simulink model "rsa_mwr2mm_core"  (R2021b)
settings: Solver=VariableStepAuto  StartTime=0.0  StopTime=simulation_time  RelTol=1e-3
values from neighbouring files (symbols this model uses):
  E = fi(hex2dec("4741"),0,max_n_bit,0)    [mwr2mm_init.m]    (also in rsa_mwr2mm_init.m)
  K = fi(mod((4)^max_n_bit,double(N)),0,max_n_bit,0)    [mwr2mm_init.m]    (also in rsa_mwr2mm_init.m)
  M = fi(hex2dec("2f76"),0,max_n_bit,0)    [mwr2mm_init.m]    (also in rsa_mwr2mm_init.m)
  max_n_bit = 16    [mwr2mm_init.m]    (also in rsa_mwr2mm_init.m)
  N = fi(hex2dec("8167"),0,max_n_bit,0)    [mwr2mm_init.m]    (also in rsa_mwr2mm_init.m)
  number_of_pe = ceil((max_n_bit+1)/word_length)    [mwr2mm_init.m]    (also in rsa_mwr2mm_init.m)
  ts = 1/fs    (= 4e-09)    [mwr2mm_init.m]    (also in rsa_mwr2mm_init.m)
  word_length = 4    [mwr2mm_init.m]    (also in rsa_mwr2mm_init.m)
libraries: xbsIndex_r4 x206
(part 1 of 2)
settings Model: Creator=HosseinBehehsti  LastModifiedBy=sysgen

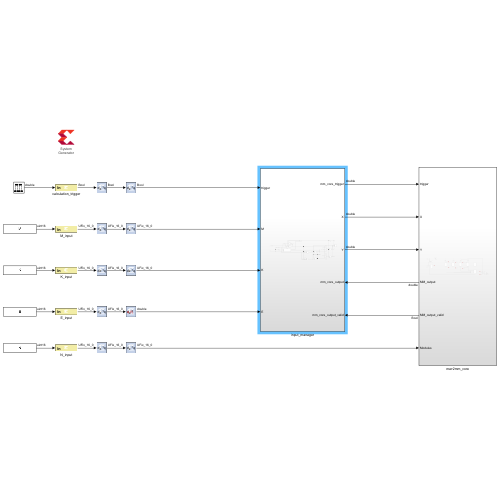
[thumbnail: Simulink's stored preview of the top-level diagram]
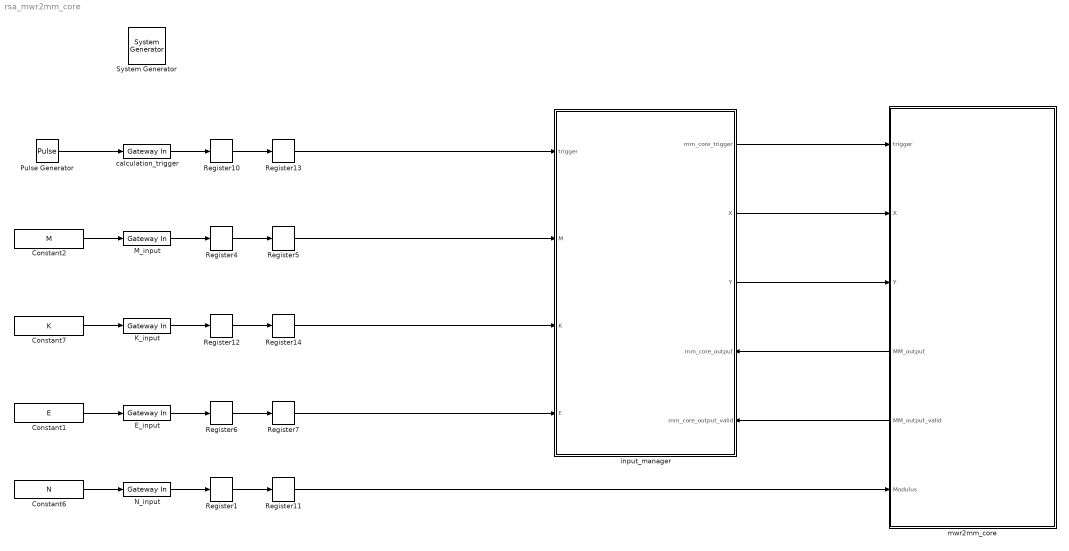
== system rsa_mwr2mm_core ==
  " System Generator" : xbsIndex_r4/ System Generator  Tag=genX  xilinxfamily=kintex7  part=xc7k325t  speed=-2  package=ffg676  synthesis_tool=Vivado  clock_wrapper=Clock Enables  directory=./netlist  proj_type=Vivado  Synth_file=Vivado Synthesis Defaults  Impl_file=Vivado Implementation Defaults  testbench=off  simulink_period=ts  sysclk_period=ts*1e9  dcm_input_clock_period=10  incr_netlist=off  trim_vbits=Everywhere in SubSystem  dbl_ovrd=According to Block Masks  core_generation=According to Block Masks  run_coregen=off  deprecated_control=off  eval_field=0  block_type=sysgen
  Constant1 : Constant  Value=E
  Constant2 : Constant  Value=M
  Constant6 : Constant  Value=N
  Constant7 : Constant  Value=K
  E_input : xbsIndex_r4/Gateway In  gui_display_data_type=Fixed-point  arith_type=Unsigned  n_bits=max_n_bit  bin_pt=0  preci_type=Single  exp_width=8  frac_width=24  rows=1  columns=1  quantization="Round  (unbiased: +/- Inf)"  overflow=Saturate  period=ts  UseAsADC=off  ADCChannel='1'  interface=None  automatic_assignment=on  address_offset=hex2dec('00')  intf_name=''  intf_description=''  default_value=0  timing_constraint=None  locs_specified=off  LOCs={}  io_standard={}  inherit_from_input=off  hdl_port=on  dbl_ovrd=off  block_type=gatewayin
  K_input : xbsIndex_r4/Gateway In  gui_display_data_type=Fixed-point  arith_type=Unsigned  n_bits=max_n_bit  bin_pt=0  preci_type=Single  exp_width=8  frac_width=24  rows=1  columns=1  quantization="Round  (unbiased: +/- Inf)"  overflow=Saturate  period=ts  UseAsADC=off  ADCChannel='1'  interface=None  automatic_assignment=on  address_offset=hex2dec('00')  intf_name=''  intf_description=''  default_value=0  timing_constraint=None  locs_specified=off  LOCs={}  io_standard={}  inherit_from_input=off  hdl_port=on  dbl_ovrd=off  block_type=gatewayin
  M_input : xbsIndex_r4/Gateway In  gui_display_data_type=Fixed-point  arith_type=Unsigned  n_bits=max_n_bit  bin_pt=0  preci_type=Single  exp_width=8  frac_width=24  rows=1  columns=1  quantization="Round  (unbiased: +/- Inf)"  overflow=Saturate  period=ts  UseAsADC=off  ADCChannel='1'  interface=None  automatic_assignment=on  address_offset=hex2dec('00')  intf_name=''  intf_description=''  default_value=0  timing_constraint=None  locs_specified=off  LOCs={}  io_standard={}  inherit_from_input=off  hdl_port=on  dbl_ovrd=off  block_type=gatewayin
  N_input : xbsIndex_r4/Gateway In  gui_display_data_type=Fixed-point  arith_type=Unsigned  n_bits=max_n_bit  bin_pt=0  preci_type=Single  exp_width=8  frac_width=24  rows=1  columns=1  quantization="Round  (unbiased: +/- Inf)"  overflow=Saturate  period=ts  UseAsADC=off  ADCChannel='1'  interface=None  automatic_assignment=on  address_offset=hex2dec('00')  intf_name=''  intf_description=''  default_value=0  timing_constraint=None  locs_specified=off  LOCs={}  io_standard={}  inherit_from_input=off  hdl_port=on  dbl_ovrd=off  block_type=gatewayin
  Pulse Generator : DiscretePulseGenerator  Period=10000  PhaseDelay=30  SampleTime=ts
  Register{1,4..7,10..14} (10 alike) : xbsIndex_r4/Register  init=0  rst=off  en=off  dbl_ovrd=off  block_type=register
  calculation_trigger : xbsIndex_r4/Gateway In  gui_display_data_type=Boolean  arith_type=Boolean  n_bits=16  bin_pt=14  preci_type=Single  exp_width=8  frac_width=24  rows=1  columns=1  quantization="Round  (unbiased: +/- Inf)"  overflow=Saturate  period=ts  UseAsADC=off  ADCChannel='1'  interface=None  automatic_assignment=on  address_offset=hex2dec('00')  intf_name=''  intf_description=''  default_value=0  timing_constraint=None  locs_specified=off  LOCs={}  io_standard={}  inherit_from_input=off  hdl_port=on  dbl_ovrd=off  block_type=gatewayin
  input_manager : Subsystem
      settings: PortSchema="{\"entries\":[{\"content\":{\"sides\":[{\"content\":{\"connectorIds\":[\"In1\",\"In2\",\"In3\",\"In4\"]},\"type\":\"ConnectorPlacement.EquallySpacedRectSide\",\"uuid\":\"5fbe749b-9735-44fd-a2bb-776500a26cf7\"},{\"content\":{\"connectorIds\":[\"Out1\",\"Out2\",\"Out3\",\"In5\",\"In6\"],\"side\":\"RIGHT\"},\"type\":\"ConnectorPlacement.EquallySpacedRectSide\",\"uuid\":\"76eb6fff-7389-4eb3-99ce-2472142167d3\"},{\"content\":{\"connectorIds\":[],\"side\":\"TOP\"},\"type\":\"ConnectorPlacement.EquallySpacedRectSide\",\"uuid\":\"3dd7521d-ec81-483b-a940-2bc8a970d0b7\"}]},\"type\":\"ConnectorPlacement.EquallySpacedConnector\",\"uuid\":\"ad526796-1480-458f-ab98-8695681b9dff\"}],\"packageUris\":[\"http://schema.mathworks.com/mf0/Connector/R2020b\"],\"version\":\"1.0\"}"
  mwr2mm_core : Subsystem
      settings: PortSchema="{\"entries\":[{\"content\":{\"sides\":[{\"content\":{\"connectorIds\":[\"In1\",\"In2\",\"In3\",\"Out1\",\"Out2\",\"In4\"]},\"type\":\"ConnectorPlacement.EquallySpacedRectSide\",\"uuid\":\"3849742e-47e7-45e9-813d-75e7ec89f679\"},{\"content\":{\"connectorIds\":[],\"side\":\"RIGHT\"},\"type\":\"ConnectorPlacement.EquallySpacedRectSide\",\"uuid\":\"56ecc40d-88ec-4579-a1b5-d15bded2ad6c\"},{\"content\":{\"connectorIds\":[],\"side\":\"TOP\"},\"type\":\"ConnectorPlacement.EquallySpacedRectSide\",\"uuid\":\"95912069-9c19-4eb9-99de-47b6cc07ccbf\"}]},\"type\":\"ConnectorPlacement.EquallySpacedConnector\",\"uuid\":\"0eef9a1f-cfa8-4a5c-bd29-08fde97e02e9\"}],\"packageUris\":[\"http://schema.mathworks.com/mf0/Connector/R2020b\"],\"version\":\"1.0\"}"
  wires:
  Register4/1 -> Register5/1
  M_input/1 -> Register4/1
  E_input/1 -> Register6/1
  Register6/1 -> Register7/1
  Register10/1 -> Register13/1
  calculation_trigger/1 -> Register10/1
  Constant1/1 -> E_input/1
  Constant2/1 -> M_input/1
  Pulse Generator/1 -> calculation_trigger/1
  Constant6/1 -> N_input/1
  Register1/1 -> Register11/1
  N_input/1 -> Register1/1
  K_input/1 -> Register12/1
  Register12/1 -> Register14/1
  Constant7/1 -> K_input/1
  Register11/1 -> mwr2mm_core/4(Modulus)
  Register5/1 -> input_manager/2(M)
  Register14/1 -> input_manager/3(K)
  input_manager/2(X) -> mwr2mm_core/2(X)
  input_manager/3(Y) -> mwr2mm_core/3(Y)
  Register13/1 -> input_manager/1(trigger)
  Register7/1 -> input_manager/4(E)
  input_manager/1(mm_core_trigger) -> mwr2mm_core/1(trigger)
  mwr2mm_core/1(MM_output) -> input_manager/5(mm_core_output)
  mwr2mm_core/2(MM_output_valid) -> input_manager/6(mm_core_output_valid)

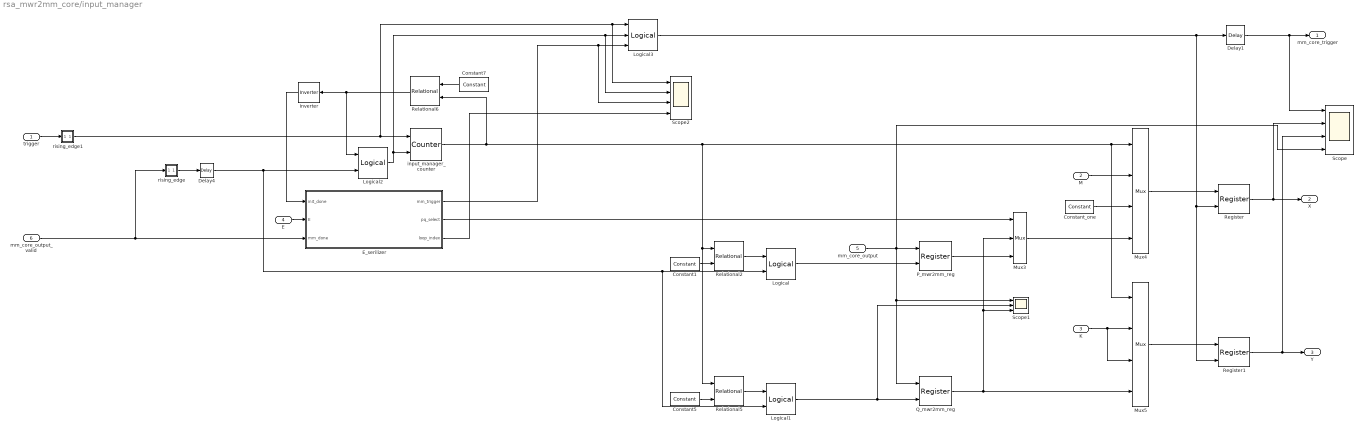
== system rsa_mwr2mm_core/input_manager ==
  trigger : Inport
  M : Inport  Port=2
  K : Inport  Port=3
  E : Inport  Port=4
  mm_core_output : Inport  Port=5
  mm_core_output_valid : Inport  Port=6
  Constant1 : xbsIndex_r4/Constant  const=0  gui_display_data_type=Fixed-point  arith_type=Unsigned  n_bits=2  bin_pt=0  preci_type=Single  exp_width=8  frac_width=24  explicit_period=off  period=1  equ=P=C  opselect=C  inp2=PCIN>>17  opr=+  inp1=P  carry=CIN  dbl_ovrd=off  block_type=constant
  Constant5 : xbsIndex_r4/Constant  const=0  gui_display_data_type=Fixed-point  arith_type=Unsigned  n_bits=2  bin_pt=0  preci_type=Single  exp_width=8  frac_width=24  explicit_period=off  period=1  equ=P=C  opselect=C  inp2=PCIN>>17  opr=+  inp1=P  carry=CIN  dbl_ovrd=off  block_type=constant
  Constant7 : xbsIndex_r4/Constant  const=2  gui_display_data_type=Fixed-point  arith_type=Unsigned  n_bits=2  bin_pt=0  preci_type=Single  exp_width=8  frac_width=24  explicit_period=off  period=1  equ=P=C  opselect=C  inp2=PCIN>>17  opr=+  inp1=P  carry=CIN  dbl_ovrd=off  block_type=constant
  Constant_one : xbsIndex_r4/Constant  const=1.0  gui_display_data_type=Fixed-point  arith_type=Unsigned  n_bits=max_n_bit  bin_pt=0  preci_type=Single  exp_width=8  frac_width=24  explicit_period=off  period=1  equ=P=C  opselect=C  inp2=PCIN>>17  opr=+  inp1=P  carry=CIN  dbl_ovrd=off  block_type=constant
  Delay1 : xbsIndex_r4/Delay  rst=off  infoeditControl=Selection of Reset will increase slice count due to use of real FFs and instead of SRLs  en=off  latency=4  reg_retiming=off  dbl_ovrd=off  block_type=delay
  Delay4 : xbsIndex_r4/Delay  rst=off  infoeditControl=Selection of Reset will increase slice count due to use of real FFs and instead of SRLs  en=off  latency=11  reg_retiming=off  dbl_ovrd=off  block_type=delay
  E_serilizer : Subsystem
  Inverter : xbsIndex_r4/Inverter  en=off  latency=1  dbl_ovrd=off  block_type=inv
  Logical : xbsIndex_r4/Logical  logical_function=AND  inputs=2  en=off  latency=1  precision=Full  arith_type=Unsigned  n_bits=16  bin_pt=0  align_bp=on  dbl_ovrd=off  block_type=logical
  Logical1 : xbsIndex_r4/Logical  logical_function=AND  inputs=2  en=off  latency=1  precision=Full  arith_type=Unsigned  n_bits=16  bin_pt=0  align_bp=on  dbl_ovrd=off  block_type=logical
  Logical2 : xbsIndex_r4/Logical  logical_function=AND  inputs=2  en=off  latency=0  precision=Full  arith_type=Unsigned  n_bits=16  bin_pt=0  align_bp=on  dbl_ovrd=off  block_type=logical
  Logical3 : xbsIndex_r4/Logical  logical_function=OR  inputs=3  en=off  latency=0  precision=Full  arith_type=Unsigned  n_bits=16  bin_pt=0  align_bp=on  dbl_ovrd=off  block_type=logical
  Mux3 : xbsIndex_r4/Mux  inputs=2  en=off  latency=0  precision=Full  arith_type=Unsigned  n_bits=16  bin_pt=14  quantization=Truncate  overflow=Wrap  dbl_ovrd=off  block_type=mux
  Mux4 : xbsIndex_r4/Mux  inputs=3  en=off  latency=1  precision=Full  arith_type=Unsigned  n_bits=16  bin_pt=14  quantization=Truncate  overflow=Wrap  dbl_ovrd=off  block_type=mux
  Mux5 : xbsIndex_r4/Mux  inputs=3  en=off  latency=1  precision=Full  arith_type=Unsigned  n_bits=16  bin_pt=14  quantization=Truncate  overflow=Wrap  dbl_ovrd=off  block_type=mux
  P_mwr2mm_reg : xbsIndex_r4/Register  init=0  rst=off  en=on  dbl_ovrd=off  block_type=register
  Q_mwr2mm_reg : xbsIndex_r4/Register  init=0  rst=off  en=on  dbl_ovrd=off  block_type=register
  Register : xbsIndex_r4/Register  init=0  rst=off  en=on  dbl_ovrd=off  block_type=register
  Register1 : xbsIndex_r4/Register  init=0  rst=off  en=on  dbl_ovrd=off  block_type=register
  Relational2 : xbsIndex_r4/Relational  mode=a=b  op_type=Bool  en=off  latency=0  dbl_ovrd=off  block_type=relational
  Relational5 : xbsIndex_r4/Relational  mode=a!=b  op_type=Bool  en=off  latency=0  dbl_ovrd=off  block_type=relational
  Relational6 : xbsIndex_r4/Relational  mode=a!=b  op_type=Bool  en=off  latency=0  dbl_ovrd=off  block_type=relational
  Scope : Scope  NumInputPorts=4
  Scope1 : Scope  NumInputPorts=3
  Scope2 : Scope  NumInputPorts=4
  input_manager_counter : xbsIndex_r4/Counter  cnt_type=Count Limited  cnt_to=2  operation=Up  start_count=0  cnt_by_val=1  arith_type=Unsigned  n_bits=2  bin_pt=0  load_pin=off  rst=on  en=on  explicit_period=off  period=1  use_behavioral_HDL=off  implementation=Fabric  dbl_ovrd=off  block_type=counter
  rising_edge : Subsystem
  rising_edge1 : Subsystem
  mm_core_trigger : Outport
  X : Outport  Port=2
  Y : Outport  Port=3
  wires:
  E_serilizer/2(pq_select) -> Mux3/1
  Q_mwr2mm_reg/1 -> Mux5/4, Scope1/3, Mux3/2
  P_mwr2mm_reg/1 -> Mux3/3
  mm_core_output/1 -> Q_mwr2mm_reg/1, Scope1/1, Scope/4, P_mwr2mm_reg/1
  mm_core_output_valid/1 -> rising_edge/1(input), E_serilizer/3(mm_done)
  Relational2/1 -> Logical/1
  Constant1/1 -> Relational2/2
  Logical/1 -> P_mwr2mm_reg/2
  trigger/1 -> rising_edge1/1(input)
  rising_edge1/1(redge) -> Scope2/1, Logical3/1, input_manager_counter/1
  E_serilizer/1(mm_trigger) -> Scope2/3, Logical3/3
  Constant5/1 -> Relational5/2
  Relational5/1 -> Logical1/1
  Logical1/1 -> Scope1/2, Q_mwr2mm_reg/2
  E/1 -> E_serilizer/2(E)
  Constant7/1 -> Relational6/1
  Logical2/1 -> Scope2/2, Logical3/2, input_manager_counter/2
  Relational6/1 -> Logical2/1, Inverter/1
  Inverter/1 -> E_serilizer/1(init_done)
  input_manager_counter/1 -> Relational6/2, Mux5/1, Mux4/1, Relational5/1, Relational2/1
  rising_edge/1(redge) -> Delay4/1
  Delay4/1 -> Logical2/2, Logical1/2, Logical/2
  Register/1 -> Scope/2, X/1
  Register1/1 -> Scope/3, Y/1
  Delay1/1 -> Scope/1, mm_core_trigger/1
  M/1 -> Mux4/2
  Mux4/1 -> Register/1
  Mux5/1 -> Register1/1
  K/1 -> Mux5/3, Mux5/2
  Constant_one/1 -> Mux4/3
  Mux3/1 -> Mux4/4
  Logical3/1 -> Register/2, Register1/2, Delay1/1
  E_serilizer/3(loop_index) -> Scope2/4

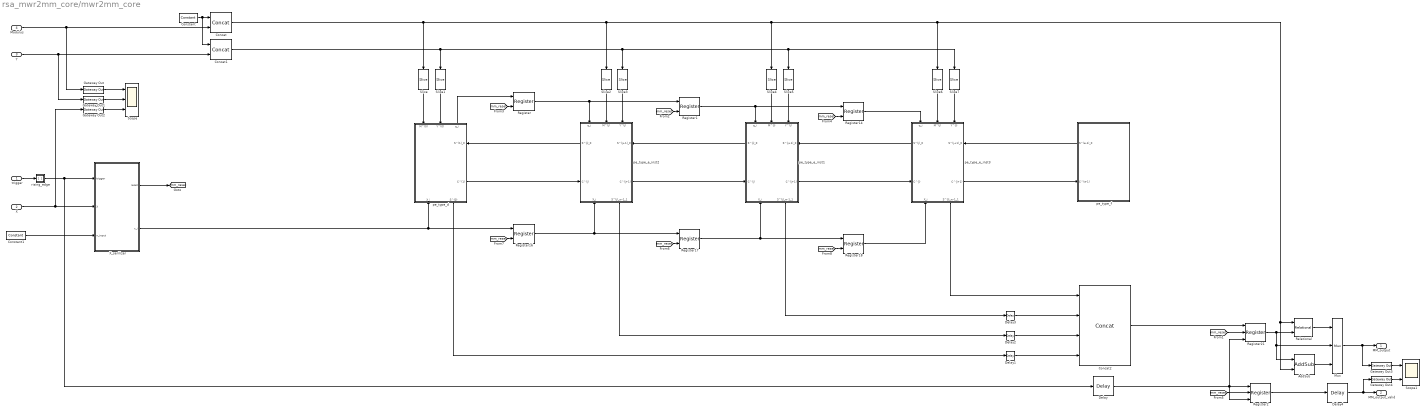
== system rsa_mwr2mm_core/mwr2mm_core ==
  trigger : Inport
  X : Inport  Port=2
  Y : Inport  Port=3
  Modulus : Inport  Port=4
  AddSub : xbsIndex_r4/AddSub  mode=Subtraction  use_carryin=off  use_carryout=off  en=off  latency=1  precision=User Defined  arith_type=Unsigned  n_bits=max_n_bit  bin_pt=0  quantization="Round  (unbiased: +/- Inf)"  overflow=Saturate  use_behavioral_HDL=off  hw_selection=Fabric  pipelined=off  dbl_ovrd=off  block_type=addsub
  Concat : xbsIndex_r4/Concat  num_inputs=2  dbl_ovrd=off  block_type=concat
  Concat1 : xbsIndex_r4/Concat  num_inputs=2  dbl_ovrd=off  block_type=concat
  Concat2 : xbsIndex_r4/Concat  num_inputs=4  dbl_ovrd=off  block_type=concat
  Constant : xbsIndex_r4/Constant  const=0  gui_display_data_type=Fixed-point  arith_type=Unsigned  n_bits=word_length  bin_pt=0  preci_type=Single  exp_width=8  frac_width=24  explicit_period=off  period=1  equ=P=C  opselect=C  inp2=PCIN>>17  opr=+  inp1=P  carry=CIN  dbl_ovrd=off  block_type=constant
  Constant1 : xbsIndex_r4/Constant  const=max_n_bit-1  gui_display_data_type=Fixed-point  arith_type=Unsigned  n_bits=ceil(log2(max_n_bit))  bin_pt=0  preci_type=Single  exp_width=8  frac_width=24  explicit_period=on  period=ts  equ=P=C  opselect=C  inp2=PCIN>>17  opr=+  inp1=P  carry=CIN  dbl_ovrd=off  block_type=constant
  Delay : xbsIndex_r4/Delay  rst=off  infoeditControl=Selection of Reset will increase slice count due to use of real FFs and instead of SRLs  en=off  latency=max_n_bit+number_of_pe+5  reg_retiming=off  dbl_ovrd=off  block_type=delay
  Delay1 : xbsIndex_r4/Delay  rst=off  infoeditControl=Selection of Reset will increase slice count due to use of real FFs and instead of SRLs  en=off  latency=3  reg_retiming=off  dbl_ovrd=off  block_type=delay
  Delay2 : xbsIndex_r4/Delay  rst=off  infoeditControl=Selection of Reset will increase slice count due to use of real FFs and instead of SRLs  en=off  latency=2  reg_retiming=off  dbl_ovrd=off  block_type=delay
  Delay3 : xbsIndex_r4/Delay  rst=off  infoeditControl=Selection of Reset will increase slice count due to use of real FFs and instead of SRLs  en=off  latency=1  reg_retiming=off  dbl_ovrd=off  block_type=delay
  Delay4 : xbsIndex_r4/Delay  rst=off  infoeditControl=Selection of Reset will increase slice count due to use of real FFs and instead of SRLs  en=off  latency=3  reg_retiming=off  dbl_ovrd=off  block_type=delay
  Gateway Out{,1..4} (5 alike) : xbsIndex_r4/Gateway Out  inherit_from_input=off  hdl_port=off  rows=1  columns=1  UseAsDAC=off  DACChannel='1'  interface=None  automatic_assignment=on  address_offset=hex2dec('00')  intf_name=''  intf_description=''  timing_constraint=None  locs_specified=off  LOCs={}  io_standard={}  block_type=gatewayout
  Mux : xbsIndex_r4/Mux  inputs=2  en=off  latency=1  precision=Full  arith_type=Unsigned  n_bits=16  bin_pt=14  quantization=Truncate  overflow=Wrap  dbl_ovrd=off  block_type=mux
  Register{,1,14,16..18} (6 alike) : xbsIndex_r4/Register  init=0  rst=on  en=off  dbl_ovrd=off  block_type=register
  Register2 : xbsIndex_r4/Register  init=0  rst=on  en=on  dbl_ovrd=off  block_type=register
  Register21 : xbsIndex_r4/Register  init=0  rst=on  en=on  dbl_ovrd=off  block_type=register
  Relational : xbsIndex_r4/Relational  mode=a<b  op_type=Bool  en=off  latency=1  dbl_ovrd=off  block_type=relational
  Scope : Scope  NumInputPorts=3
  Scope1 : Scope  NumInputPorts=2
  Slice : xbsIndex_r4/Slice  nbits=word_length  boolean_output=off  mode=Lower Bit Location + Width  bit1=0  base1=MSB of Input  bit0=0  base0=LSB of Input  dbl_ovrd=off  block_type=slice
  Slice1 : xbsIndex_r4/Slice  nbits=word_length  boolean_output=off  mode=Lower Bit Location + Width  bit1=0  base1=MSB of Input  bit0=0  base0=LSB of Input  dbl_ovrd=off  block_type=slice
  Slice2 : xbsIndex_r4/Slice  nbits=word_length  boolean_output=off  mode=Lower Bit Location + Width  bit1=0  base1=MSB of Input  bit0=1*word_length  base0=LSB of Input  dbl_ovrd=off  block_type=slice
  Slice3 : xbsIndex_r4/Slice  nbits=word_length  boolean_output=off  mode=Lower Bit Location + Width  bit1=0  base1=MSB of Input  bit0=1*word_length  base0=LSB of Input  dbl_ovrd=off  block_type=slice
  Slice4 : xbsIndex_r4/Slice  nbits=word_length  boolean_output=off  mode=Lower Bit Location + Width  bit1=0  base1=MSB of Input  bit0=2*word_length  base0=LSB of Input  dbl_ovrd=off  block_type=slice
  Slice5 : xbsIndex_r4/Slice  nbits=word_length  boolean_output=off  mode=Lower Bit Location + Width  bit1=0  base1=MSB of Input  bit0=2*word_length  base0=LSB of Input  dbl_ovrd=off  block_type=slice
  Slice6 : xbsIndex_r4/Slice  nbits=word_length  boolean_output=off  mode=Lower Bit Location + Width  bit1=0  base1=MSB of Input  bit0=3*word_length  base0=LSB of Input  dbl_ovrd=off  block_type=slice
  Slice7 : xbsIndex_r4/Slice  nbits=word_length  boolean_output=off  mode=Lower Bit Location + Width  bit1=0  base1=MSB of Input  bit0=3*word_length  base0=LSB of Input  dbl_ovrd=off  block_type=slice
  X_serilizer : Subsystem
  pe_type_d : Subsystem
      settings: PortSchema="{\"entries\":[{\"content\":{\"sides\":[{\"content\":{\"connectorIds\":[]},\"type\":\"ConnectorPlacement.EquallySpacedRectSide\",\"uuid\":\"139fe22c-bad5-4a8c-bb4f-0e4abe8a2134\"},{\"content\":{\"connectorIds\":[\"In4\",\"Out1\"],\"side\":\"RIGHT\"},\"type\":\"ConnectorPlacement.EquallySpacedRectSide\",\"uuid\":\"0caa1206-8436-46b5-be2a-5ee3acf33157\"},{\"content\":{\"connectorIds\":[\"In1\",\"In2\",\"Out3\"],\"side\":\"TOP\"},\"type\":\"ConnectorPlacement.EquallySpacedRectSide\",\"uuid\":\"0f19409c-37a1-4e1f-8a36-d56d656a29ed\"},{\"content\":{\"connectorIds\":[\"In3\",\"Out2\"],\"side\":\"BOTTOM\"},\"type\":\"ConnectorPlacement.EquallySpacedRectSide\",\"uuid\":\"3eb4fdbb-82ed-4bb4-bb3d-1ea670375199\"}]},\"type\":\"ConnectorPlacement.EquallySpacedConnector\",\"uuid\":\"2e2112f8-b3e9-4cf9-af24-9d5d119acc0c\"}],\"packageUris\":[\"http://schema.mathworks.com/mf0/Connector/R2020b\"],\"version\":\"1.0\"}"
  pe_type_e_inst1 : Subsystem
      settings: PortSchema="{\"entries\":[{\"content\":{\"sides\":[{\"content\":{\"connectorIds\":[\"Out3\",\"In1\"]},\"type\":\"ConnectorPlacement.EquallySpacedRectSide\",\"uuid\":\"7c8435b2-413b-47b3-86e2-fbe621383b46\"},{\"content\":{\"connectorIds\":[\"In6\",\"Out1\"],\"side\":\"RIGHT\"},\"type\":\"ConnectorPlacement.EquallySpacedRectSide\",\"uuid\":\"f6a32e17-79c6-4fcd-9120-5459a6da7349\"},{\"content\":{\"connectorIds\":[\"In2\",\"In3\",\"In4\"],\"side\":\"TOP\"},\"type\":\"ConnectorPlacement.EquallySpacedRectSide\",\"uuid\":\"72801329-e094-46db-be09-4f98df807717\"},{\"content\":{\"connectorIds\":[\"In5\",\"Out2\"],\"side\":\"BOTTOM\"},\"type\":\"ConnectorPlacement.EquallySpacedRectSide\",\"uuid\":\"81172500-9a38-48f4-98da-a2165838752d\"}]},\"type\":\"ConnectorPlacement.EquallySpacedConnector\",\"uuid\":\"de64cd8a-ab75-41df-a3d4-83ece8cdbbe2\"}],\"packageUris\":[\"http://schema.mathworks.com/mf0/Connector/R2020b\"],\"version\":\"1.0\"}"
  pe_type_e_inst2 : Subsystem
      settings: PortSchema="{\"entries\":[{\"content\":{\"sides\":[{\"content\":{\"connectorIds\":[\"Out3\",\"In1\"]},\"type\":\"ConnectorPlacement.EquallySpacedRectSide\",\"uuid\":\"7c8435b2-413b-47b3-86e2-fbe621383b46\"},{\"content\":{\"connectorIds\":[\"In6\",\"Out1\"],\"side\":\"RIGHT\"},\"type\":\"ConnectorPlacement.EquallySpacedRectSide\",\"uuid\":\"f6a32e17-79c6-4fcd-9120-5459a6da7349\"},{\"content\":{\"connectorIds\":[\"In2\",\"In3\",\"In4\"],\"side\":\"TOP\"},\"type\":\"ConnectorPlacement.EquallySpacedRectSide\",\"uuid\":\"72801329-e094-46db-be09-4f98df807717\"},{\"content\":{\"connectorIds\":[\"In5\",\"Out2\"],\"side\":\"BOTTOM\"},\"type\":\"ConnectorPlacement.EquallySpacedRectSide\",\"uuid\":\"81172500-9a38-48f4-98da-a2165838752d\"}]},\"type\":\"ConnectorPlacement.EquallySpacedConnector\",\"uuid\":\"de64cd8a-ab75-41df-a3d4-83ece8cdbbe2\"}],\"packageUris\":[\"http://schema.mathworks.com/mf0/Connector/R2020b\"],\"version\":\"1.0\"}"
  pe_type_e_inst3 : Subsystem
      settings: PortSchema="{\"entries\":[{\"content\":{\"sides\":[{\"content\":{\"connectorIds\":[\"Out3\",\"In1\"]},\"type\":\"ConnectorPlacement.EquallySpacedRectSide\",\"uuid\":\"7c8435b2-413b-47b3-86e2-fbe621383b46\"},{\"content\":{\"connectorIds\":[\"In6\",\"Out1\"],\"side\":\"RIGHT\"},\"type\":\"ConnectorPlacement.EquallySpacedRectSide\",\"uuid\":\"f6a32e17-79c6-4fcd-9120-5459a6da7349\"},{\"content\":{\"connectorIds\":[\"In2\",\"In3\",\"In4\"],\"side\":\"TOP\"},\"type\":\"ConnectorPlacement.EquallySpacedRectSide\",\"uuid\":\"72801329-e094-46db-be09-4f98df807717\"},{\"content\":{\"connectorIds\":[\"In5\",\"Out2\"],\"side\":\"BOTTOM\"},\"type\":\"ConnectorPlacement.EquallySpacedRectSide\",\"uuid\":\"81172500-9a38-48f4-98da-a2165838752d\"}]},\"type\":\"ConnectorPlacement.EquallySpacedConnector\",\"uuid\":\"de64cd8a-ab75-41df-a3d4-83ece8cdbbe2\"}],\"packageUris\":[\"http://schema.mathworks.com/mf0/Connector/R2020b\"],\"version\":\"1.0\"}"
  pe_type_f : Subsystem
      settings: PortSchema="{\"entries\":[{\"content\":{\"sides\":[{\"content\":{\"connectorIds\":[\"Out1\",\"In1\"]},\"type\":\"ConnectorPlacement.EquallySpacedRectSide\",\"uuid\":\"7c8435b2-413b-47b3-86e2-fbe621383b46\"},{\"content\":{\"connectorIds\":[],\"side\":\"RIGHT\"},\"type\":\"ConnectorPlacement.EquallySpacedRectSide\",\"uuid\":\"f6a32e17-79c6-4fcd-9120-5459a6da7349\"},{\"content\":{\"connectorIds\":[],\"side\":\"TOP\"},\"type\":\"ConnectorPlacement.EquallySpacedRectSide\",\"uuid\":\"72801329-e094-46db-be09-4f98df807717\"},{\"content\":{\"connectorIds\":[],\"side\":\"BOTTOM\"},\"type\":\"ConnectorPlacement.EquallySpacedRectSide\",\"uuid\":\"86ccfa13-264b-4b98-8cad-be21ce563201\"}]},\"type\":\"ConnectorPlacement.EquallySpacedConnector\",\"uuid\":\"de64cd8a-ab75-41df-a3d4-83ece8cdbbe2\"}],\"packageUris\":[\"http://schema.mathworks.com/mf0/Connector/R2020b\"],\"version\":\"1.0\"}"
  rising_edge : Subsystem
  MM_output : Outport
  MM_output_valid : Outport  Port=2
  tag scope: mm_reset=global
  wires:
  pe_type_d/2(S^(0)) -> Delay1/1
  [mm_reset] -> Register14/2
  pe_type_e_inst1/1(C^(j+1)) -> pe_type_e_inst3/1(C^(j))
  pe_type_d/1(C^(1)) -> pe_type_e_inst2/1(C^(j))
  Register16/1 -> pe_type_e_inst2/5(X_i), Register17/1
  Delay3/1 -> Concat2/2
  Register17/1 -> pe_type_e_inst1/5(X_i), Register18/1
  Register18/1 -> pe_type_e_inst3/5(X_i)
  Concat/1 -> Slice/1, Slice2/1, Slice4/1, Slice6/1, AddSub/2, Relational/1
  pe_type_e_inst2/1(C^(j+1)) -> pe_type_e_inst1/1(C^(j))
  X_serilizer/2(x_i) -> pe_type_d/3(X_i), Register16/1
  Register21/1 -> AddSub/1, Mux/2, Relational/2
  pe_type_e_inst1/2(S^(j)_w-1_1) -> Delay3/1
  pe_type_e_inst3/2(S^(j)_w-1_1) -> Concat2/1
  pe_type_e_inst2/2(S^(j)_w-1_1) -> Delay2/1
  Slice2/1 -> pe_type_e_inst2/3(M^(j))
  AddSub/1 -> Mux/3
  pe_type_f/1(S^(e-1)_0) -> pe_type_e_inst3/6(S^(j+1)_0)
  pe_type_d/3(q_i) -> Register/1
  [mm_reset] -> Register21/2
  trigger/1 -> rising_edge/1(input)
  Slice6/1 -> pe_type_e_inst3/3(M^(j))
  Concat1/1 -> Slice1/1, Slice3/1, Slice5/1, Slice7/1
  pe_type_e_inst3/3(S^(j)_0) -> pe_type_e_inst1/6(S^(j+1)_0)
  Register1/1 -> pe_type_e_inst1/2(q_i), Register14/1
  [mm_reset] -> Register18/2
  pe_type_e_inst2/3(S^(j)_0) -> pe_type_d/4(S^(1)_0)
  Delay2/1 -> Concat2/3
  Constant/1 -> Concat1/1, Concat/1
  Register14/1 -> pe_type_e_inst3/2(q_i)
  [mm_reset] -> Register/2
  Delay1/1 -> Concat2/4
  X_serilizer/1(reset) -> [mm_reset]
  [mm_reset] -> Register17/2
  pe_type_e_inst1/3(S^(j)_0) -> pe_type_e_inst2/6(S^(j+1)_0)
  [mm_reset] -> Register1/2
  Slice7/1 -> pe_type_e_inst3/4(Y^(j))
  Slice/1 -> pe_type_d/1(M^(0))
  Register/1 -> pe_type_e_inst2/2(q_i), Register1/1
  [mm_reset] -> Register16/2
  Slice5/1 -> pe_type_e_inst1/4(Y^(j))
  X/1 -> Gateway Out2/1, X_serilizer/2(X)
  Relational/1 -> Mux/1
  Slice1/1 -> pe_type_d/2(Y^(0))
  Slice3/1 -> pe_type_e_inst2/4(Y^(j))
  rising_edge/1(redge) -> Delay/1, X_serilizer/1(trigger)
  Delay/1 -> Register2/3, Register2/1, Register21/3
  pe_type_e_inst3/1(C^(j+1)) -> pe_type_f/1(C^(e-1))
  Y/1 -> Gateway Out1/1, Concat1/2
  Slice4/1 -> pe_type_e_inst1/3(M^(j))
  Concat2/1 -> Register21/1
  Mux/1 -> Gateway Out3/1, MM_output/1
  Modulus/1 -> Gateway Out/1, Concat/2
  [mm_reset] -> Register2/2
  Register2/1 -> Delay4/1
  Delay4/1 -> MM_output_valid/1, Gateway Out4/1
  Constant1/1 -> X_serilizer/3(n_input)
  Gateway Out/1 -> Scope/1
  Gateway Out1/1 -> Scope/2
  Gateway Out2/1 -> Scope/3
  Gateway Out3/1 -> Scope1/1
  Gateway Out4/1 -> Scope1/2

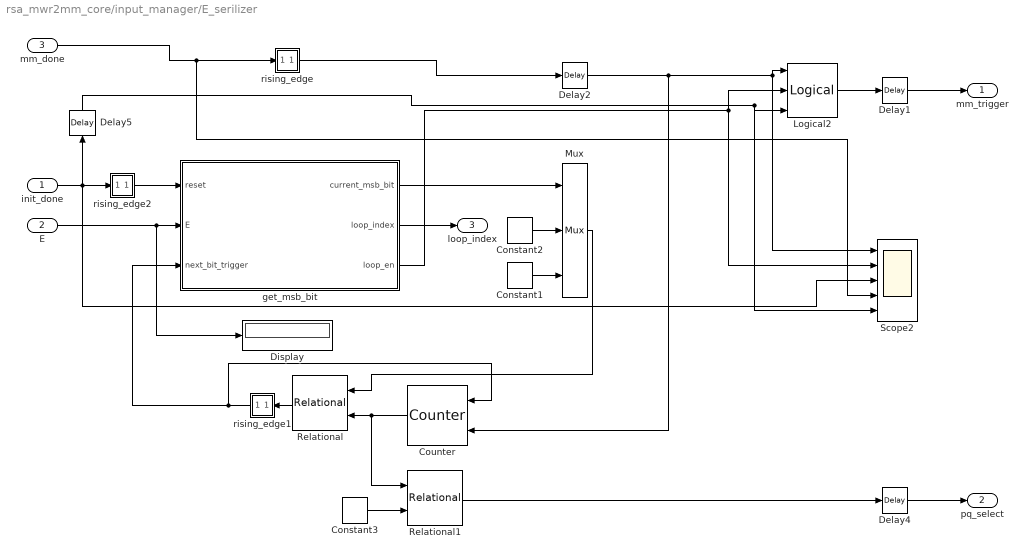
== system rsa_mwr2mm_core/input_manager/E_serilizer ==
  init_done : Inport
  E : Inport  Port=2
  mm_done : Inport  Port=3
  Constant1 : xbsIndex_r4/Constant  const=2  gui_display_data_type=Fixed-point  arith_type=Unsigned  n_bits=2  bin_pt=0  preci_type=Single  exp_width=8  frac_width=24  explicit_period=off  period=1  equ=P=C  opselect=C  inp2=PCIN>>17  opr=+  inp1=P  carry=CIN  dbl_ovrd=off  block_type=constant
  Constant2 : xbsIndex_r4/Constant  const=1  gui_display_data_type=Fixed-point  arith_type=Unsigned  n_bits=2  bin_pt=0  preci_type=Single  exp_width=8  frac_width=24  explicit_period=off  period=1  equ=P=C  opselect=C  inp2=PCIN>>17  opr=+  inp1=P  carry=CIN  dbl_ovrd=off  block_type=constant
  Constant3 : xbsIndex_r4/Constant  const=1  gui_display_data_type=Fixed-point  arith_type=Unsigned  n_bits=2  bin_pt=0  preci_type=Single  exp_width=8  frac_width=24  explicit_period=off  period=1  equ=P=C  opselect=C  inp2=PCIN>>17  opr=+  inp1=P  carry=CIN  dbl_ovrd=off  block_type=constant
  Counter : xbsIndex_r4/Counter  cnt_type=Free Running  cnt_to=Inf  operation=Up  start_count=0  cnt_by_val=1  arith_type=Unsigned  n_bits=8  bin_pt=0  load_pin=off  rst=on  en=on  explicit_period=off  period=1  use_behavioral_HDL=off  implementation=Fabric  dbl_ovrd=off  block_type=counter
  Delay1 : xbsIndex_r4/Delay  rst=off  infoeditControl=Selection of Reset will increase slice count due to use of real FFs and instead of SRLs  en=off  latency=5  reg_retiming=off  dbl_ovrd=off  block_type=delay
  Delay2 : xbsIndex_r4/Delay  rst=off  infoeditControl=Selection of Reset will increase slice count due to use of real FFs and instead of SRLs  en=off  latency=10  reg_retiming=off  dbl_ovrd=off  block_type=delay
  Delay4 : xbsIndex_r4/Delay  rst=off  infoeditControl=Selection of Reset will increase slice count due to use of real FFs and instead of SRLs  en=off  latency=5  reg_retiming=off  dbl_ovrd=off  block_type=delay
  Delay5 : xbsIndex_r4/Delay  rst=off  infoeditControl=Selection of Reset will increase slice count due to use of real FFs and instead of SRLs  en=off  latency=5  reg_retiming=off  dbl_ovrd=off  block_type=delay
  Display : Display
      settings: Format=binary (Stored Integer)
  Logical2 : xbsIndex_r4/Logical  logical_function=AND  inputs=3  en=off  latency=1  precision=Full  arith_type=Unsigned  n_bits=16  bin_pt=0  align_bp=on  dbl_ovrd=off  block_type=logical
  Mux : xbsIndex_r4/Mux  inputs=2  en=off  latency=1  precision=Full  arith_type=Unsigned  n_bits=16  bin_pt=14  quantization=Truncate  overflow=Wrap  dbl_ovrd=off  block_type=mux
  Relational : xbsIndex_r4/Relational  mode=a=b  op_type=Bool  en=off  latency=1  dbl_ovrd=off  block_type=relational
  Relational1 : xbsIndex_r4/Relational  mode=a=b  op_type=Bool  en=off  latency=1  dbl_ovrd=off  block_type=relational
  Scope2 : Scope  NumInputPorts=5
  get_msb_bit : Subsystem
  rising_edge : Subsystem
  rising_edge1 : Subsystem
  rising_edge2 : Subsystem
  mm_trigger : Outport
  pq_select : Outport  Port=2
  loop_index : Outport  Port=3
  wires:
  mm_done/1 -> Scope2/4, rising_edge/1(input)
  Relational1/1 -> Delay4/1
  Delay1/1 -> mm_trigger/1
  init_done/1 -> Scope2/3, rising_edge2/1(input), Delay5/1
  E/1 -> Display/1, get_msb_bit/2(E)
  rising_edge/1(redge) -> Delay2/1
  rising_edge2/1(redge) -> get_msb_bit/1(reset)
  Delay5/1 -> Scope2/5, Logical2/3
  get_msb_bit/1(current_msb_bit) -> Mux/1
  Constant2/1 -> Mux/2
  Constant1/1 -> Mux/3
  Counter/1 -> Relational1/1, Relational/2
  Mux/1 -> Relational/1
  Relational/1 -> rising_edge1/1(input)
  rising_edge1/1(redge) -> get_msb_bit/3(next_bit_trigger), Counter/1
  Constant3/1 -> Relational1/2
  Logical2/1 -> Delay1/1
  get_msb_bit/3(loop_en) -> Logical2/2, Scope2/2
  get_msb_bit/2(loop_index) -> loop_index/1
  Delay4/1 -> pq_select/1
  Delay2/1 -> Scope2/1, Logical2/1, Counter/2

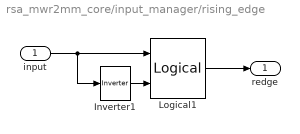
== system rsa_mwr2mm_core/input_manager/rising_edge ==
  input : Inport
  Inverter1 : xbsIndex_r4/Inverter  en=off  latency=1  dbl_ovrd=off  block_type=inv
  Logical1 : xbsIndex_r4/Logical  logical_function=AND  inputs=2  en=off  latency=0  precision=Full  arith_type=Unsigned  n_bits=16  bin_pt=0  align_bp=on  dbl_ovrd=off  block_type=logical
  redge : Outport
  wires:
  Inverter1/1 -> Logical1/2
  input/1 -> Inverter1/1, Logical1/1
  Logical1/1 -> redge/1

== system rsa_mwr2mm_core/input_manager/rising_edge1 ==
  input : Inport
  Inverter1 : xbsIndex_r4/Inverter  en=off  latency=1  dbl_ovrd=off  block_type=inv
  Logical1 : xbsIndex_r4/Logical  logical_function=AND  inputs=2  en=off  latency=0  precision=Full  arith_type=Unsigned  n_bits=16  bin_pt=0  align_bp=on  dbl_ovrd=off  block_type=logical
  redge : Outport
  wires:
  Logical1/1 -> redge/1
  input/1 -> Logical1/1, Inverter1/1
  Inverter1/1 -> Logical1/2

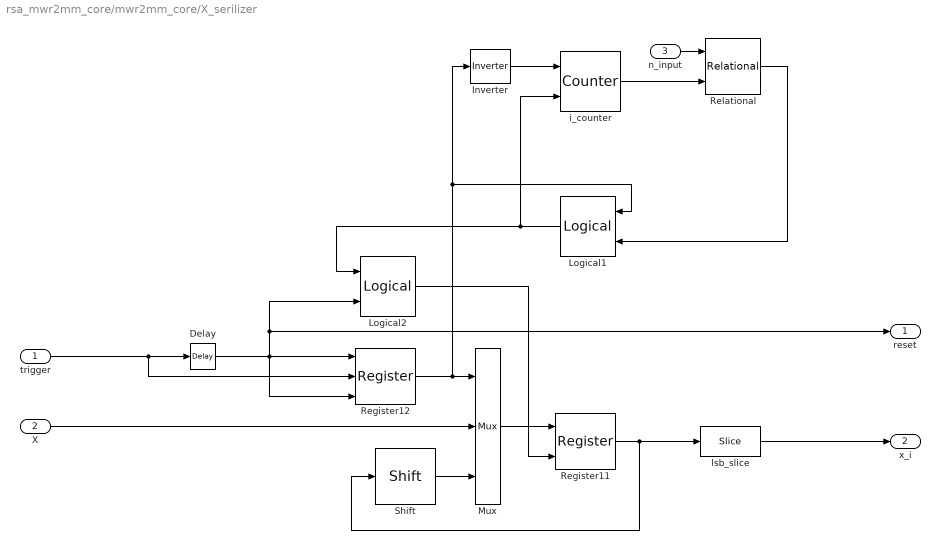
== system rsa_mwr2mm_core/mwr2mm_core/X_serilizer ==
  trigger : Inport
  X : Inport  Port=2
  n_input : Inport  Port=3
  Delay : xbsIndex_r4/Delay  rst=off  infoeditControl=Selection of Reset will increase slice count due to use of real FFs and instead of SRLs  en=off  latency=5  reg_retiming=off  dbl_ovrd=off  block_type=delay
  Inverter : xbsIndex_r4/Inverter  en=off  latency=0  dbl_ovrd=off  block_type=inv
  Logical1 : xbsIndex_r4/Logical  logical_function=AND  inputs=2  en=off  latency=0  precision=Full  arith_type=Unsigned  n_bits=16  bin_pt=0  align_bp=on  dbl_ovrd=off  block_type=logical
  Logical2 : xbsIndex_r4/Logical  logical_function=OR  inputs=2  en=off  latency=0  precision=Full  arith_type=Unsigned  n_bits=16  bin_pt=0  align_bp=on  dbl_ovrd=off  block_type=logical
  Mux : xbsIndex_r4/Mux  inputs=2  en=off  latency=0  precision=Full  arith_type=Unsigned  n_bits=16  bin_pt=14  quantization=Truncate  overflow=Wrap  dbl_ovrd=off  block_type=mux
  Register11 : xbsIndex_r4/Register  init=0  rst=off  en=on  dbl_ovrd=off  block_type=register
  Register12 : xbsIndex_r4/Register  init=0  rst=on  en=on  dbl_ovrd=off  block_type=register
  Relational : xbsIndex_r4/Relational  mode=a>=b  op_type=Bool  en=off  latency=0  dbl_ovrd=off  block_type=relational
  Shift : xbsIndex_r4/Shift  shift_dir=Right  shift_bits=1  en=off  latency=0  precision=Full  arith_type="Signed  (2's comp)"  n_bits=16  bin_pt=14  quantization=Truncate  overflow=Wrap  dbl_ovrd=off  block_type=shift
  i_counter : xbsIndex_r4/Counter  cnt_type=Free Running  cnt_to=Inf  operation=Up  start_count=0  cnt_by_val=1  arith_type=Unsigned  n_bits=ceil(log2(max_n_bit))+1  bin_pt=0  load_pin=off  rst=on  en=on  explicit_period=off  period=1  use_behavioral_HDL=off  implementation=Fabric  dbl_ovrd=off  block_type=counter
  lsb_slice : xbsIndex_r4/Slice  nbits=1  boolean_output=on  mode=Lower Bit Location + Width  bit1=0  base1=MSB of Input  bit0=0  base0=LSB of Input  dbl_ovrd=off  block_type=slice
  reset : Outport
  x_i : Outport  Port=2
  wires:
  Register12/1 -> Inverter/1, Logical1/1, Mux/1
  Mux/1 -> Register11/1
  Shift/1 -> Mux/3
  Register11/1 -> Shift/1, lsb_slice/1
  Relational/1 -> Logical1/2
  i_counter/1 -> Relational/2
  Logical2/1 -> Register11/2
  n_input/1 -> Relational/1
  X/1 -> Mux/2
  Logical1/1 -> i_counter/2, Logical2/1
  Inverter/1 -> i_counter/1
  trigger/1 -> Register12/2, Delay/1
  lsb_slice/1 -> x_i/1
  Delay/1 -> Register12/3, reset/1, Logical2/2, Register12/1

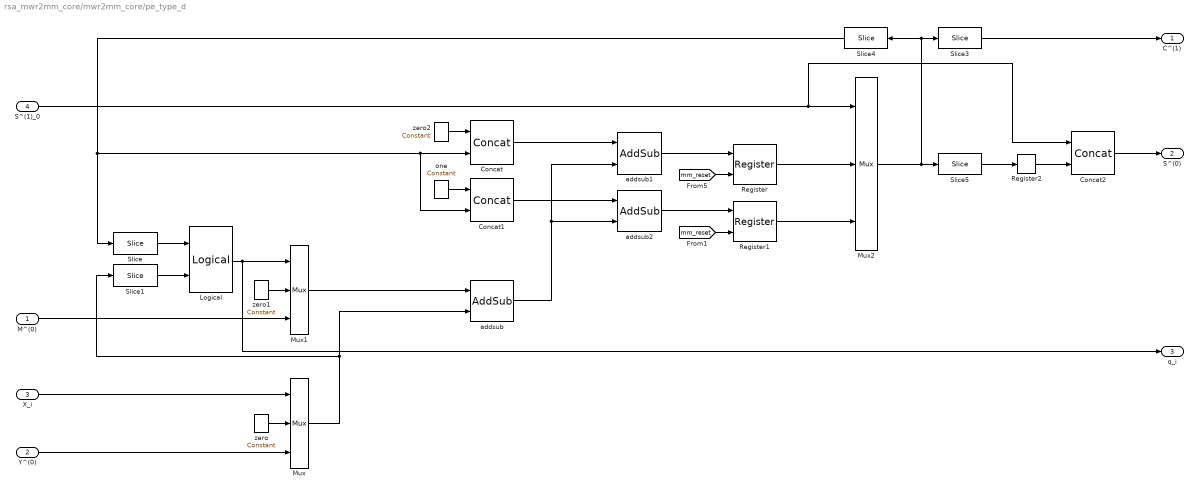
== system rsa_mwr2mm_core/mwr2mm_core/pe_type_d ==
  M^(0) : Inport
  Y^(0) : Inport  Port=2
  X_i : Inport  Port=3
  S^(1)_0 : Inport  Port=4
  Concat : xbsIndex_r4/Concat  num_inputs=2  dbl_ovrd=off  block_type=concat
  Concat1 : xbsIndex_r4/Concat  num_inputs=2  dbl_ovrd=off  block_type=concat
  Concat2 : xbsIndex_r4/Concat  num_inputs=2  dbl_ovrd=off  block_type=concat
  Logical : xbsIndex_r4/Logical  logical_function=XOR  inputs=2  en=off  latency=0  precision=Full  arith_type=Unsigned  n_bits=16  bin_pt=0  align_bp=on  dbl_ovrd=off  block_type=logical
  Mux : xbsIndex_r4/Mux  inputs=2  en=off  latency=0  precision=Full  arith_type=Unsigned  n_bits=16  bin_pt=14  quantization=Truncate  overflow=Wrap  dbl_ovrd=off  block_type=mux
  Mux1 : xbsIndex_r4/Mux  inputs=2  en=off  latency=0  precision=Full  arith_type=Unsigned  n_bits=16  bin_pt=14  quantization=Truncate  overflow=Wrap  dbl_ovrd=off  block_type=mux
  Mux2 : xbsIndex_r4/Mux  inputs=2  en=off  latency=0  precision=Full  arith_type=Unsigned  n_bits=16  bin_pt=14  quantization=Truncate  overflow=Wrap  dbl_ovrd=off  block_type=mux
  Register : xbsIndex_r4/Register  init=0  rst=on  en=off  dbl_ovrd=off  block_type=register
  Register1 : xbsIndex_r4/Register  init=0  rst=on  en=off  dbl_ovrd=off  block_type=register
  Register2 : xbsIndex_r4/Register  init=0  rst=off  en=off  dbl_ovrd=off  block_type=register
  Slice : xbsIndex_r4/Slice  nbits=1  boolean_output=on  mode=Lower Bit Location + Width  bit1=0  base1=MSB of Input  bit0=0  base0=LSB of Input  dbl_ovrd=off  block_type=slice
  Slice1 : xbsIndex_r4/Slice  nbits=1  boolean_output=on  mode=Lower Bit Location + Width  bit1=0  base1=MSB of Input  bit0=0  base0=LSB of Input  dbl_ovrd=off  block_type=slice
  Slice3 : xbsIndex_r4/Slice  nbits=2  boolean_output=off  mode=Lower Bit Location + Width  bit1=0  base1=MSB of Input  bit0=word_length  base0=LSB of Input  dbl_ovrd=off  block_type=slice
  Slice4 : xbsIndex_r4/Slice  nbits=word_length-1  boolean_output=off  mode=Lower Bit Location + Width  bit1=0  base1=MSB of Input  bit0=1  base0=LSB of Input  dbl_ovrd=off  block_type=slice
  Slice5 : xbsIndex_r4/Slice  nbits=word_length-1  boolean_output=off  mode=Lower Bit Location + Width  bit1=0  base1=MSB of Input  bit0=1  base0=LSB of Input  dbl_ovrd=off  block_type=slice
  addsub : xbsIndex_r4/AddSub  mode=Addition  use_carryin=off  use_carryout=off  en=off  latency=0  precision=User Defined  arith_type=Unsigned  n_bits=word_length+1  bin_pt=0  quantization="Round  (unbiased: +/- Inf)"  overflow=Saturate  use_behavioral_HDL=off  hw_selection=Fabric  pipelined=off  dbl_ovrd=off  block_type=addsub
  addsub1 : xbsIndex_r4/AddSub  mode=Addition  use_carryin=off  use_carryout=off  en=off  latency=0  precision=User Defined  arith_type=Unsigned  n_bits=word_length+2  bin_pt=0  quantization="Round  (unbiased: +/- Inf)"  overflow=Saturate  use_behavioral_HDL=off  hw_selection=Fabric  pipelined=off  dbl_ovrd=off  block_type=addsub
  addsub2 : xbsIndex_r4/AddSub  mode=Addition  use_carryin=off  use_carryout=off  en=off  latency=0  precision=User Defined  arith_type=Unsigned  n_bits=word_length+2  bin_pt=0  quantization="Round  (unbiased: +/- Inf)"  overflow=Saturate  use_behavioral_HDL=off  hw_selection=Fabric  pipelined=off  dbl_ovrd=off  block_type=addsub
  one : xbsIndex_r4/Constant  const=1  gui_display_data_type=Fixed-point  arith_type=Unsigned  n_bits=1  bin_pt=0  preci_type=Single  exp_width=8  frac_width=24  explicit_period=off  period=1  equ=P=C  opselect=C  inp2=PCIN>>17  opr=+  inp1=P  carry=CIN  dbl_ovrd=off  block_type=constant
  zero : xbsIndex_r4/Constant  const=0  gui_display_data_type=Fixed-point  arith_type=Unsigned  n_bits=1  bin_pt=0  preci_type=Single  exp_width=8  frac_width=24  explicit_period=off  period=1  equ=P=C  opselect=C  inp2=PCIN>>17  opr=+  inp1=P  carry=CIN  dbl_ovrd=off  block_type=constant
  zero1 : xbsIndex_r4/Constant  const=0  gui_display_data_type=Fixed-point  arith_type=Unsigned  n_bits=1  bin_pt=0  preci_type=Single  exp_width=8  frac_width=24  explicit_period=off  period=1  equ=P=C  opselect=C  inp2=PCIN>>17  opr=+  inp1=P  carry=CIN  dbl_ovrd=off  block_type=constant
  zero2 : xbsIndex_r4/Constant  const=0  gui_display_data_type=Fixed-point  arith_type=Unsigned  n_bits=1  bin_pt=0  preci_type=Single  exp_width=8  frac_width=24  explicit_period=off  period=1  equ=P=C  opselect=C  inp2=PCIN>>17  opr=+  inp1=P  carry=CIN  dbl_ovrd=off  block_type=constant
  C^(1) : Outport
  S^(0) : Outport  Port=2
  q_i : Outport  Port=3
  wires:
  Logical/1 -> q_i/1, Mux1/1
  Mux2/1 -> Slice5/1, Slice3/1, Slice4/1
  addsub2/1 -> Register1/1
  addsub1/1 -> Register/1
  Concat1/1 -> addsub2/1
  Concat/1 -> addsub1/1
  one/1 -> Concat1/1
  Mux1/1 -> addsub/1
  Slice/1 -> Logical/1
  Mux/1 -> Slice1/1, addsub/2
  Slice1/1 -> Logical/2
  zero1/1 -> Mux1/2
  Y^(0)/1 -> Mux/3
  zero/1 -> Mux/2
  M^(0)/1 -> Mux1/3
  X_i/1 -> Mux/1
  Register1/1 -> Mux2/3
  Slice3/1 -> C^(1)/1
  [mm_reset] -> Register/2
  [mm_reset] -> Register1/2
  Slice5/1 -> Register2/1
  Concat2/1 -> S^(0)/1
  Register2/1 -> Concat2/2
  Register/1 -> Mux2/2
  zero2/1 -> Concat/1
  Slice4/1 -> Slice/1, Concat1/2, Concat/2
  addsub/1 -> addsub2/2, addsub1/2
  S^(1)_0/1 -> Mux2/1, Concat2/1

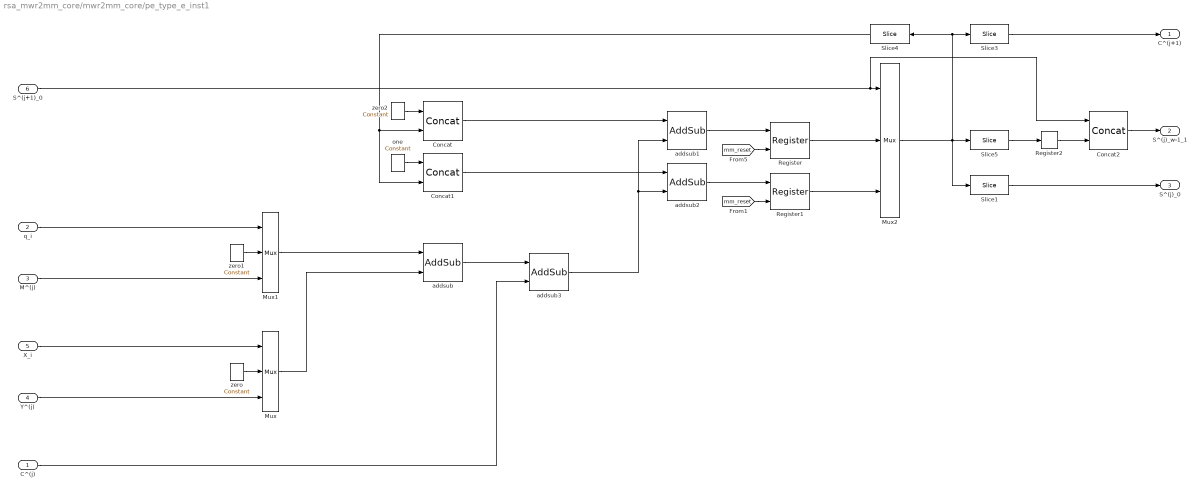
== system rsa_mwr2mm_core/mwr2mm_core/pe_type_e_inst1 ==
  C^(j) : Inport
  q_i : Inport  Port=2
  M^(j) : Inport  Port=3
  Y^(j) : Inport  Port=4
  X_i : Inport  Port=5
  S^(j+1)_0 : Inport  Port=6
  Concat : xbsIndex_r4/Concat  num_inputs=2  dbl_ovrd=off  block_type=concat
  Concat1 : xbsIndex_r4/Concat  num_inputs=2  dbl_ovrd=off  block_type=concat
  Concat2 : xbsIndex_r4/Concat  num_inputs=2  dbl_ovrd=off  block_type=concat
  Mux : xbsIndex_r4/Mux  inputs=2  en=off  latency=0  precision=Full  arith_type=Unsigned  n_bits=16  bin_pt=14  quantization=Truncate  overflow=Wrap  dbl_ovrd=off  block_type=mux
  Mux1 : xbsIndex_r4/Mux  inputs=2  en=off  latency=0  precision=Full  arith_type=Unsigned  n_bits=16  bin_pt=14  quantization=Truncate  overflow=Wrap  dbl_ovrd=off  block_type=mux
  Mux2 : xbsIndex_r4/Mux  inputs=2  en=off  latency=0  precision=Full  arith_type=Unsigned  n_bits=16  bin_pt=14  quantization=Truncate  overflow=Wrap  dbl_ovrd=off  block_type=mux
  Register : xbsIndex_r4/Register  init=0  rst=on  en=off  dbl_ovrd=off  block_type=register
  Register1 : xbsIndex_r4/Register  init=0  rst=on  en=off  dbl_ovrd=off  block_type=register
  Register2 : xbsIndex_r4/Register  init=0  rst=off  en=off  dbl_ovrd=off  block_type=register
  Slice1 : xbsIndex_r4/Slice  nbits=word_length-1  boolean_output=on  mode=Lower Bit Location + Width  bit1=0  base1=MSB of Input  bit0=0  base0=LSB of Input  dbl_ovrd=off  block_type=slice
  Slice3 : xbsIndex_r4/Slice  nbits=2  boolean_output=off  mode=Lower Bit Location + Width  bit1=0  base1=MSB of Input  bit0=word_length  base0=LSB of Input  dbl_ovrd=off  block_type=slice
  Slice4 : xbsIndex_r4/Slice  nbits=word_length-1  boolean_output=off  mode=Lower Bit Location + Width  bit1=0  base1=MSB of Input  bit0=1  base0=LSB of Input  dbl_ovrd=off  block_type=slice
  Slice5 : xbsIndex_r4/Slice  nbits=word_length-1  boolean_output=off  mode=Lower Bit Location + Width  bit1=0  base1=MSB of Input  bit0=1  base0=LSB of Input  dbl_ovrd=off  block_type=slice
  addsub : xbsIndex_r4/AddSub  mode=Addition  use_carryin=off  use_carryout=off  en=off  latency=0  precision=User Defined  arith_type=Unsigned  n_bits=word_length+1  bin_pt=0  quantization="Round  (unbiased: +/- Inf)"  overflow=Saturate  use_behavioral_HDL=off  hw_selection=Fabric  pipelined=on  dbl_ovrd=off  block_type=addsub
  addsub1 : xbsIndex_r4/AddSub  mode=Addition  use_carryin=off  use_carryout=off  en=off  latency=0  precision=User Defined  arith_type=Unsigned  n_bits=word_length+2  bin_pt=0  quantization="Round  (unbiased: +/- Inf)"  overflow=Saturate  use_behavioral_HDL=off  hw_selection=Fabric  pipelined=on  dbl_ovrd=off  block_type=addsub
  addsub2 : xbsIndex_r4/AddSub  mode=Addition  use_carryin=off  use_carryout=off  en=off  latency=0  precision=User Defined  arith_type=Unsigned  n_bits=word_length+2  bin_pt=0  quantization="Round  (unbiased: +/- Inf)"  overflow=Saturate  use_behavioral_HDL=off  hw_selection=Fabric  pipelined=on  dbl_ovrd=off  block_type=addsub
  addsub3 : xbsIndex_r4/AddSub  mode=Addition  use_carryin=off  use_carryout=off  en=off  latency=0  precision=User Defined  arith_type=Unsigned  n_bits=word_length+2  bin_pt=0  quantization="Round  (unbiased: +/- Inf)"  overflow=Saturate  use_behavioral_HDL=off  hw_selection=Fabric  pipelined=on  dbl_ovrd=off  block_type=addsub
  one : xbsIndex_r4/Constant  const=1  gui_display_data_type=Fixed-point  arith_type=Unsigned  n_bits=1  bin_pt=0  preci_type=Single  exp_width=8  frac_width=24  explicit_period=off  period=1  equ=P=C  opselect=C  inp2=PCIN>>17  opr=+  inp1=P  carry=CIN  dbl_ovrd=off  block_type=constant
  zero : xbsIndex_r4/Constant  const=0  gui_display_data_type=Fixed-point  arith_type=Unsigned  n_bits=1  bin_pt=0  preci_type=Single  exp_width=8  frac_width=24  explicit_period=off  period=1  equ=P=C  opselect=C  inp2=PCIN>>17  opr=+  inp1=P  carry=CIN  dbl_ovrd=off  block_type=constant
  zero1 : xbsIndex_r4/Constant  const=0  gui_display_data_type=Fixed-point  arith_type=Unsigned  n_bits=1  bin_pt=0  preci_type=Single  exp_width=8  frac_width=24  explicit_period=off  period=1  equ=P=C  opselect=C  inp2=PCIN>>17  opr=+  inp1=P  carry=CIN  dbl_ovrd=off  block_type=constant
  zero2 : xbsIndex_r4/Constant  const=0  gui_display_data_type=Fixed-point  arith_type=Unsigned  n_bits=1  bin_pt=0  preci_type=Single  exp_width=8  frac_width=24  explicit_period=off  period=1  equ=P=C  opselect=C  inp2=PCIN>>17  opr=+  inp1=P  carry=CIN  dbl_ovrd=off  block_type=constant
  C^(j+1) : Outport
  S^(j)_w-1_1 : Outport  Port=2
  S^(j)_0 : Outport  Port=3
  wires:
  Slice5/1 -> Register2/1
  Register2/1 -> Concat2/2
  S^(j+1)_0/1 -> Mux2/1, Concat2/1
  Slice4/1 -> Concat1/2, Concat/2
  [mm_reset] -> Register1/2
  [mm_reset] -> Register/2
  Slice1/1 -> S^(j)_0/1
  C^(j)/1 -> addsub3/2
  addsub/1 -> addsub3/1
  Concat2/1 -> S^(j)_w-1_1/1
  q_i/1 -> Mux1/1
  Mux2/1 -> Slice3/1, Slice4/1, Slice1/1, Slice5/1
  addsub2/1 -> Register1/1
  addsub1/1 -> Register/1
  addsub3/1 -> addsub2/2, addsub1/2
  Concat1/1 -> addsub2/1
  Concat/1 -> addsub1/1
  one/1 -> Concat1/1
  zero2/1 -> Concat/1
  Mux1/1 -> addsub/1
  Mux/1 -> addsub/2
  zero1/1 -> Mux1/2
  Y^(j)/1 -> Mux/3
  zero/1 -> Mux/2
  M^(j)/1 -> Mux1/3
  X_i/1 -> Mux/1
  Register/1 -> Mux2/2
  Register1/1 -> Mux2/3
  Slice3/1 -> C^(j+1)/1

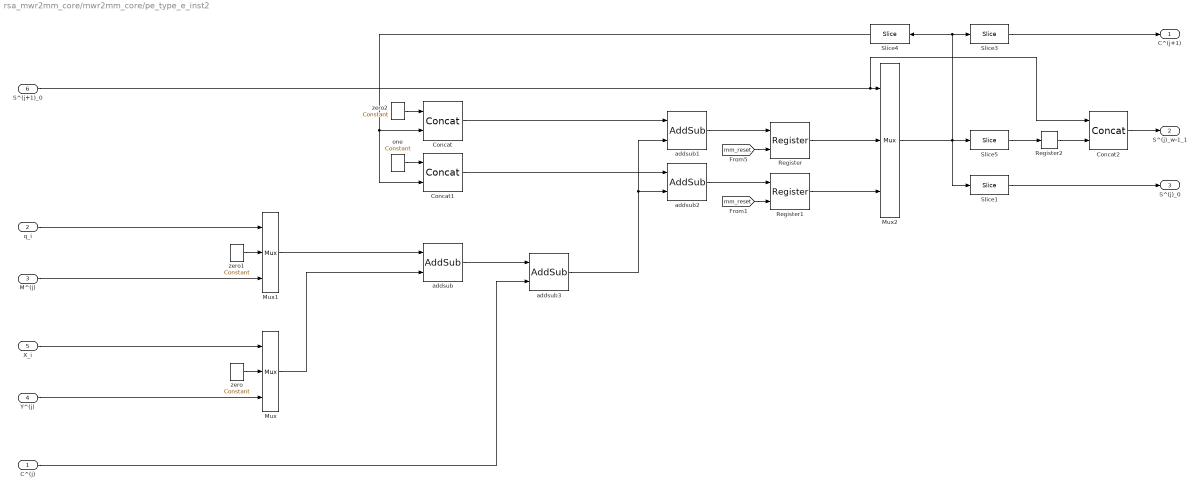
== system rsa_mwr2mm_core/mwr2mm_core/pe_type_e_inst2 ==
  C^(j) : Inport
  q_i : Inport  Port=2
  M^(j) : Inport  Port=3
  Y^(j) : Inport  Port=4
  X_i : Inport  Port=5
  S^(j+1)_0 : Inport  Port=6
  Concat : xbsIndex_r4/Concat  num_inputs=2  dbl_ovrd=off  block_type=concat
  Concat1 : xbsIndex_r4/Concat  num_inputs=2  dbl_ovrd=off  block_type=concat
  Concat2 : xbsIndex_r4/Concat  num_inputs=2  dbl_ovrd=off  block_type=concat
  Mux : xbsIndex_r4/Mux  inputs=2  en=off  latency=0  precision=Full  arith_type=Unsigned  n_bits=16  bin_pt=14  quantization=Truncate  overflow=Wrap  dbl_ovrd=off  block_type=mux
  Mux1 : xbsIndex_r4/Mux  inputs=2  en=off  latency=0  precision=Full  arith_type=Unsigned  n_bits=16  bin_pt=14  quantization=Truncate  overflow=Wrap  dbl_ovrd=off  block_type=mux
  Mux2 : xbsIndex_r4/Mux  inputs=2  en=off  latency=0  precision=Full  arith_type=Unsigned  n_bits=16  bin_pt=14  quantization=Truncate  overflow=Wrap  dbl_ovrd=off  block_type=mux
  Register : xbsIndex_r4/Register  init=0  rst=on  en=off  dbl_ovrd=off  block_type=register
  Register1 : xbsIndex_r4/Register  init=0  rst=on  en=off  dbl_ovrd=off  block_type=register
  Register2 : xbsIndex_r4/Register  init=0  rst=off  en=off  dbl_ovrd=off  block_type=register
  Slice1 : xbsIndex_r4/Slice  nbits=word_length-1  boolean_output=on  mode=Lower Bit Location + Width  bit1=0  base1=MSB of Input  bit0=0  base0=LSB of Input  dbl_ovrd=off  block_type=slice
  Slice3 : xbsIndex_r4/Slice  nbits=2  boolean_output=off  mode=Lower Bit Location + Width  bit1=0  base1=MSB of Input  bit0=word_length  base0=LSB of Input  dbl_ovrd=off  block_type=slice
  Slice4 : xbsIndex_r4/Slice  nbits=word_length-1  boolean_output=off  mode=Lower Bit Location + Width  bit1=0  base1=MSB of Input  bit0=1  base0=LSB of Input  dbl_ovrd=off  block_type=slice
  Slice5 : xbsIndex_r4/Slice  nbits=word_length-1  boolean_output=off  mode=Lower Bit Location + Width  bit1=0  base1=MSB of Input  bit0=1  base0=LSB of Input  dbl_ovrd=off  block_type=slice
  addsub : xbsIndex_r4/AddSub  mode=Addition  use_carryin=off  use_carryout=off  en=off  latency=0  precision=User Defined  arith_type=Unsigned  n_bits=word_length+1  bin_pt=0  quantization="Round  (unbiased: +/- Inf)"  overflow=Saturate  use_behavioral_HDL=off  hw_selection=Fabric  pipelined=on  dbl_ovrd=off  block_type=addsub
  addsub1 : xbsIndex_r4/AddSub  mode=Addition  use_carryin=off  use_carryout=off  en=off  latency=0  precision=User Defined  arith_type=Unsigned  n_bits=word_length+2  bin_pt=0  quantization="Round  (unbiased: +/- Inf)"  overflow=Saturate  use_behavioral_HDL=off  hw_selection=Fabric  pipelined=on  dbl_ovrd=off  block_type=addsub
  addsub2 : xbsIndex_r4/AddSub  mode=Addition  use_carryin=off  use_carryout=off  en=off  latency=0  precision=User Defined  arith_type=Unsigned  n_bits=word_length+2  bin_pt=0  quantization="Round  (unbiased: +/- Inf)"  overflow=Saturate  use_behavioral_HDL=off  hw_selection=Fabric  pipelined=on  dbl_ovrd=off  block_type=addsub
  addsub3 : xbsIndex_r4/AddSub  mode=Addition  use_carryin=off  use_carryout=off  en=off  latency=0  precision=User Defined  arith_type=Unsigned  n_bits=word_length+2  bin_pt=0  quantization="Round  (unbiased: +/- Inf)"  overflow=Saturate  use_behavioral_HDL=off  hw_selection=Fabric  pipelined=on  dbl_ovrd=off  block_type=addsub
  one : xbsIndex_r4/Constant  const=1  gui_display_data_type=Fixed-point  arith_type=Unsigned  n_bits=1  bin_pt=0  preci_type=Single  exp_width=8  frac_width=24  explicit_period=off  period=1  equ=P=C  opselect=C  inp2=PCIN>>17  opr=+  inp1=P  carry=CIN  dbl_ovrd=off  block_type=constant
  zero : xbsIndex_r4/Constant  const=0  gui_display_data_type=Fixed-point  arith_type=Unsigned  n_bits=1  bin_pt=0  preci_type=Single  exp_width=8  frac_width=24  explicit_period=off  period=1  equ=P=C  opselect=C  inp2=PCIN>>17  opr=+  inp1=P  carry=CIN  dbl_ovrd=off  block_type=constant
  zero1 : xbsIndex_r4/Constant  const=0  gui_display_data_type=Fixed-point  arith_type=Unsigned  n_bits=1  bin_pt=0  preci_type=Single  exp_width=8  frac_width=24  explicit_period=off  period=1  equ=P=C  opselect=C  inp2=PCIN>>17  opr=+  inp1=P  carry=CIN  dbl_ovrd=off  block_type=constant
  zero2 : xbsIndex_r4/Constant  const=0  gui_display_data_type=Fixed-point  arith_type=Unsigned  n_bits=1  bin_pt=0  preci_type=Single  exp_width=8  frac_width=24  explicit_period=off  period=1  equ=P=C  opselect=C  inp2=PCIN>>17  opr=+  inp1=P  carry=CIN  dbl_ovrd=off  block_type=constant
  C^(j+1) : Outport
  S^(j)_w-1_1 : Outport  Port=2
  S^(j)_0 : Outport  Port=3
  wires:
  Slice3/1 -> C^(j+1)/1
  Register1/1 -> Mux2/3
  Register/1 -> Mux2/2
  X_i/1 -> Mux/1
  M^(j)/1 -> Mux1/3
  zero/1 -> Mux/2
  Y^(j)/1 -> Mux/3
  zero1/1 -> Mux1/2
  Mux/1 -> addsub/2
  Mux1/1 -> addsub/1
  zero2/1 -> Concat/1
  one/1 -> Concat1/1
  Concat/1 -> addsub1/1
  Concat1/1 -> addsub2/1
  addsub3/1 -> addsub1/2, addsub2/2
  addsub1/1 -> Register/1
  addsub2/1 -> Register1/1
  Mux2/1 -> Slice5/1, Slice1/1, Slice4/1, Slice3/1
  q_i/1 -> Mux1/1
  Concat2/1 -> S^(j)_w-1_1/1
  addsub/1 -> addsub3/1
  C^(j)/1 -> addsub3/2
  Slice1/1 -> S^(j)_0/1
  [mm_reset] -> Register/2
  [mm_reset] -> Register1/2
  Slice4/1 -> Concat/2, Concat1/2
  S^(j+1)_0/1 -> Concat2/1, Mux2/1
  Register2/1 -> Concat2/2
  Slice5/1 -> Register2/1
